simulink model "classd"  (R2018b)
settings: Solver=ode23tb  StartTime=0.0  StopTime=.1  MaxStep=1e-3  RelTol=1e-2
libraries: powerlib x7, simulink x1
settings Model: Creator=yaoyuli  LastModifiedBy=yaoyuli
settings SolverCC: ZeroCrossControl=DisableAll

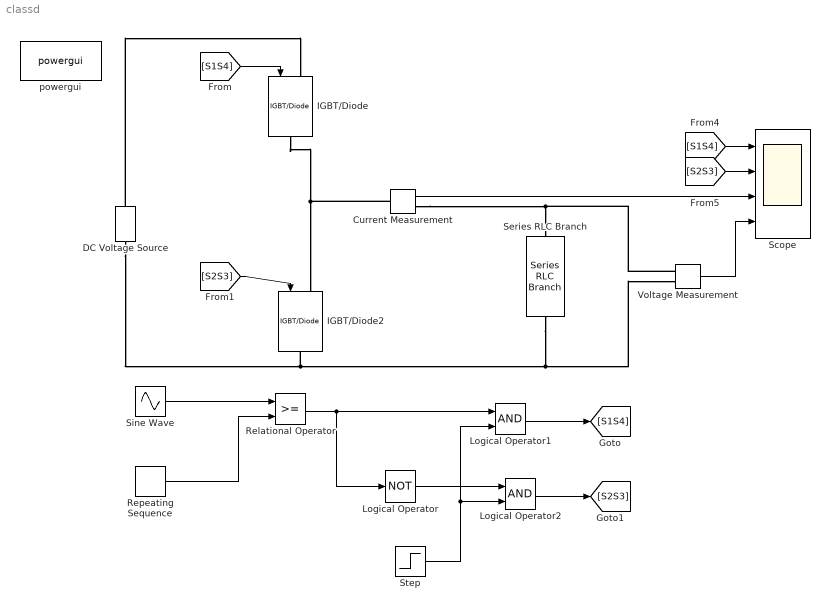
== system classd ==
  Current Measurement : powerlib/Measurements/Current Measurement  PhasorSimulation=off  OutputType=Complex  PSBequivalent=0
  DC Voltage Source : powerlib/Electrical Sources/DC Voltage Source  Amplitude=100  Measurements=None
  IGBT/Diode : powerlib/Power Electronics/IGBT//Diode  Ron=1e-3  Rs=1e5  Cs=inf  Measurements=off
  IGBT/Diode2 : powerlib/Power Electronics/IGBT//Diode  Ron=1e-3  Rs=1e5  Cs=inf  Measurements=off
  Logical Operator : Logic  Operator=NOT  AllPortsSameDT=off  OutDataTypeStr=boolean
  Logical Operator1 : Logic  AllPortsSameDT=off  OutDataTypeStr=boolean
  Logical Operator2 : Logic  AllPortsSameDT=off  OutDataTypeStr=boolean
  Relational Operator : RelationalOperator  OutDataTypeStr=boolean  RndMeth=Simplest
  Repeating Sequence : simulink/Sources/Repeating Sequence  rep_seq_t=[0 0.005/15 .01/15 .015/15 .02/15]  rep_seq_y=[0 -1 0 1 0]
  Scope : Scope  NumInputPorts=4
  Series RLC Branch : powerlib/Elements/Series RLC Branch  LConnTagsString=__new0  RConnTagsString=__new0  BranchType=RLC  Resistance=12.31  Inductance=213.49e-6  SetiL0=off  InitialCurrent=0  Capacitance=10.36e-9  Setx0=off  InitialVoltage=0  Measurements=None
  Sine Wave : Sin  Frequency=691150.383  Phase=0.523599  SampleTime=0
  Step : Step  Time=0.04  SampleTime=0
  Voltage Measurement : powerlib/Measurements/Voltage Measurement  PhasorSimulation=off  OutputType=Complex  PSBequivalent=0
  powergui : powerlib/powergui  Priority=1  SimulationMode=Continuous  SampleTime=50e-6  frequency=60  Iterations=50  frequencyindice=0  Pbase=100e6  ErrMax=1e-4  UnitsV=kV  UnitsW=MW  buscounter=0  FunctionMessages=off  echomessages=off  EnableUseOfTLC=off  CurrentSourceSwitches=off  DisableSnubberDevices=off  DisableRonSwitches=off  DisableVfSwitches=off  DisplayEquations=off  SolverType=Tustin/Backward Euler (TBE)  Interpol=off  ExternalGateDelay=off  methode=off  Ts=100  x0status=blocks  SPID=on  SwTol=0  HookPort=off  RestoreLinks=warning  ResistiveCurrentMeasurement=off  Frange=[0:2:500]  Ylog=off  Xlog=on  ShowGrid=off  save=off  variable=ZData  structure=0  ZoomFFT=off  StartTime=0.0  cycles=1  DisplayStyle=1  fundamental=60  FreqAxis=off  MaxFrequency=1000  frequencyindicesteady=1  RmsSteady=1  display=off
  wires:
  Sine Wave/1 -> Relational Operator/1
  Repeating Sequence/1 -> Relational Operator/2
  Logical Operator1/1 -> [S1S4]
  Logical Operator2/1 -> [S2S3]
  Step/1 -> Logical Operator2/2, Logical Operator1/2
  Relational Operator/1 -> Logical Operator/1, Logical Operator1/1
  Logical Operator/1 -> Logical Operator2/1
  [S1S4] -> IGBT/Diode/1
  [S2S3] -> IGBT/Diode2/1
  Current Measurement/1 -> Scope/3
  Voltage Measurement/1 -> Scope/4
  [S1S4] -> Scope/1
  [S2S3] -> Scope/2
  connections:
  IGBT/Diode/RConn1 -- IGBT/Diode2/LConn1 -- Current Measurement/LConn1
  DC Voltage Source/LConn1 -- Voltage Measurement/LConn2 -- Series RLC Branch/RConn1 -- IGBT/Diode2/RConn1
  DC Voltage Source/RConn1 -- IGBT/Diode/LConn1
  Current Measurement/RConn1 -- Voltage Measurement/LConn1 -- Series RLC Branch/LConn1
